simulink model "invPen_PID_LQR"  (R2018b)
settings: Solver=VariableStepAuto  StartTime=0.0  StopTime=20  RelTol=1e-3
libraries: simulink x4
settings Model: Creator=刘越千  LastModifiedBy=刘越千

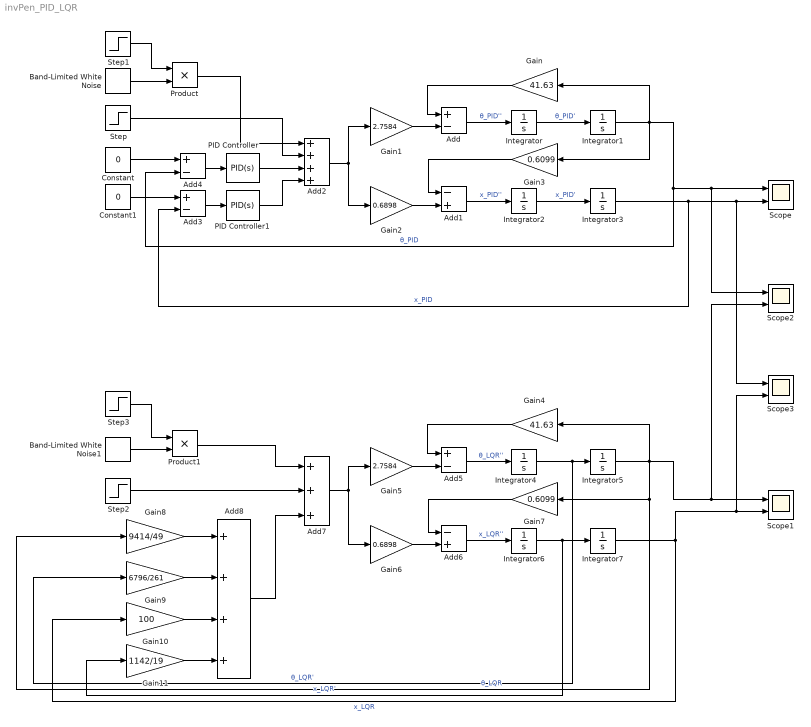
== system invPen_PID_LQR ==
  Add{,3..5} (4 alike) : Sum  Inputs=+-
  Add1 : Sum  Inputs=-+
  Add2 : Sum  Inputs=++++
  Add6 : Sum  Inputs=-+
  Add7 : Sum  Inputs=+++
  Add8 : Sum  Inputs=++++
  Band-Limited White Noise : simulink/Sources/Band-Limited White Noise  Cov=0.1  Ts=0.1  seed=[23341]
  Band-Limited White Noise1 : simulink/Sources/Band-Limited White Noise  Cov=0.1  Ts=0.1  seed=[23341]
  Constant : Constant  Value=0
  Constant1 : Constant  Value=0
  Gain : Gain  Gain=41.63
  Gain1 : Gain  Gain=2.7584
  Gain10 : Gain  Gain=100
  Gain11 : Gain  Gain=1142/19
  Gain2 : Gain  Gain=0.6898
  Gain3 : Gain  Gain=0.6099
  Gain4 : Gain  Gain=41.63
  Gain5 : Gain  Gain=2.7584
  Gain6 : Gain  Gain=0.6898
  Gain7 : Gain  Gain=0.6099
  Gain8 : Gain  Gain=9414/49
  Gain9 : Gain  Gain=6796/261
  Integrator{,2..4,6..7} (6 alike) : Integrator
  Integrator1 : Integrator  InitialCondition=0.1
  Integrator5 : Integrator  InitialCondition=0.1
  PID Controller : simulink/Continuous/PID Controller  Controller=PID  Form=Parallel  TimeDomain=Continuous-time  SampleTime=-1  IntegratorMethod=Forward Euler  FilterMethod=Forward Euler  ControllerParametersSource=internal  P=-321.380817906765  I=-1035.04229145538  D=-24.5033293148827  UseFilter=on  N=375.204412983525  TunerSelectOption=Transfer Function Based (PID Tuner App)  InitialConditionSource=internal  InitialConditionForIntegrator=0  InitialConditionForFilter=0  DifferentiatorICPrevScaledInput=0  ExternalReset=none  TrackingMode=off  Kt=1  LimitOutput=off  UpperSaturationLimit=inf  LowerSaturationLimit=-inf  LinearizeAsGain=on  AntiWindupMode=none  Kb=1  POutMin=[]  POutMax=[]  IOutMin=[]  IOutMax=[]  DOutMin=[]  DOutMax=[]  NOutMin=[]  NOutMax=[]  SumOutMin=[]  SumOutMax=[]  SaturationOutMin=[]  SaturationOutMax=[]  PParamMin=[]  PParamMax=[]  IParamMin=[]  IParamMax=[]  DParamMin=[]  DParamMax=[]  NParamMin=[]  NParamMax=[]  KbParamMin=[]  KbParamMax=[]  KtParamMin=[]  KtParamMax=[]  KbOutMin=[]  KbOutMax=[]  KtOutMin=[]  KtOutMax=[]  IntegratorOutMin=[]  IntegratorOutMax=[]  FilterOutMin=[]  FilterOutMax=[]  SumI1OutMin=[]  SumI1OutMax=[]  SumI2OutMin=[]  SumI2OutMax=[]  SumI3OutMin=[]  SumI3OutMax=[]  SumI4OutMin=[]  SumI4OutMax=[]  SumDOutMin=[]  SumDOutMax=[]  DifferentiatorOutMin=[]  DifferentiatorOutMax=[]  FilterDiffOutCoefMin=[]  FilterDiffOutCoefMax=[]  ReciprocalOutMin=[]  ReciprocalOutMax=[]  SumDenOutMin=[]  SumDenOutMax=[]  SumNumOutMin=[]  SumNumOutMax=[]  DivideOutMin=[]  DivideOutMax=[]  IntegratorContinuousStateAttributes=''  IntegratorStateMustResolveToSignalObject=off  IntegratorRTWStateStorageClass=Auto  FilterContinuousStateAttributes=''  FilterStateMustResolveToSignalObject=off  FilterRTWStateStorageClass=Auto  ParallelPVariant=InternalParameters  IdealPVariant=Disabled  IVariant=InternalParameters  DVariant=InternalParameters  IntegratorVariant=Continuous  SatVariant=Disabled  AWVariant=Passthrough  PCopyVariant=Disabled  TRVariant=Disabled  FdbkBlocksVariant=Forward  IdealPFdbkVariant=Disabled  SatFdbkVariant=Disabled  DerivativeFilterVariant=ContFilter  NVariant=InternalParameters  NCopyVariant=Disabled  FilterICVariant=InternalICsFilter  IntegratorICVariant=InternalICs  ExternalResetVariant=Disabled  TRSumVariant=Passthrough  SumFdbkVariant=Disabled  SumVariant=Sum_PID
  PID Controller1 : simulink/Continuous/PID Controller  Controller=PID  Form=Parallel  TimeDomain=Continuous-time  SampleTime=-1  IntegratorMethod=Forward Euler  FilterMethod=Forward Euler  ControllerParametersSource=internal  P=-241.711059697562  I=-56.8003532909081  D=-30.0841184690224  UseFilter=on  N=13.870046438424  TunerSelectOption=Transfer Function Based (PID Tuner App)  InitialConditionSource=internal  InitialConditionForIntegrator=0  InitialConditionForFilter=0  DifferentiatorICPrevScaledInput=0  ExternalReset=none  TrackingMode=off  Kt=1  LimitOutput=off  UpperSaturationLimit=inf  LowerSaturationLimit=-inf  LinearizeAsGain=on  AntiWindupMode=none  Kb=1  POutMin=[]  POutMax=[]  IOutMin=[]  IOutMax=[]  DOutMin=[]  DOutMax=[]  NOutMin=[]  NOutMax=[]  SumOutMin=[]  SumOutMax=[]  SaturationOutMin=[]  SaturationOutMax=[]  PParamMin=[]  PParamMax=[]  IParamMin=[]  IParamMax=[]  DParamMin=[]  DParamMax=[]  NParamMin=[]  NParamMax=[]  KbParamMin=[]  KbParamMax=[]  KtParamMin=[]  KtParamMax=[]  KbOutMin=[]  KbOutMax=[]  KtOutMin=[]  KtOutMax=[]  IntegratorOutMin=[]  IntegratorOutMax=[]  FilterOutMin=[]  FilterOutMax=[]  SumI1OutMin=[]  SumI1OutMax=[]  SumI2OutMin=[]  SumI2OutMax=[]  SumI3OutMin=[]  SumI3OutMax=[]  SumI4OutMin=[]  SumI4OutMax=[]  SumDOutMin=[]  SumDOutMax=[]  DifferentiatorOutMin=[]  DifferentiatorOutMax=[]  FilterDiffOutCoefMin=[]  FilterDiffOutCoefMax=[]  ReciprocalOutMin=[]  ReciprocalOutMax=[]  SumDenOutMin=[]  SumDenOutMax=[]  SumNumOutMin=[]  SumNumOutMax=[]  DivideOutMin=[]  DivideOutMax=[]  IntegratorContinuousStateAttributes=''  IntegratorStateMustResolveToSignalObject=off  IntegratorRTWStateStorageClass=Auto  FilterContinuousStateAttributes=''  FilterStateMustResolveToSignalObject=off  FilterRTWStateStorageClass=Auto  ParallelPVariant=InternalParameters  IdealPVariant=Disabled  IVariant=InternalParameters  DVariant=InternalParameters  IntegratorVariant=Continuous  SatVariant=Disabled  AWVariant=Passthrough  PCopyVariant=Disabled  TRVariant=Disabled  FdbkBlocksVariant=Forward  IdealPFdbkVariant=Disabled  SatFdbkVariant=Disabled  DerivativeFilterVariant=ContFilter  NVariant=InternalParameters  NCopyVariant=Disabled  FilterICVariant=InternalICsFilter  IntegratorICVariant=InternalICs  ExternalResetVariant=Disabled  TRSumVariant=Passthrough  SumFdbkVariant=Disabled  SumVariant=Sum_PID
  Product : Product
  Product1 : Product
  Scope{,1..3} (4 alike) : Scope  NumInputPorts=2
  Step : Step  Time=2  After=10  SampleTime=0
  Step1 : Step  Time=15  SampleTime=0
  Step2 : Step  Time=2  After=10  SampleTime=0
  Step3 : Step  Time=15  SampleTime=0
  wires:
  Gain11/1 -> Add8/4
  Band-Limited White Noise1/1 -> Product1/2
  Integrator7/1 -> Gain10/1, Scope3/2, Scope1/2  "x_LQR"
  Gain6/1 -> Add6/2
  Step3/1 -> Product1/1
  Add7/1 -> Gain6/1, Gain5/1
  Add8/1 -> Add7/3
  Integrator6/1 -> Gain11/1, Integrator7/1  "x_LQR'"
  Integrator5/1 -> Gain8/1, Gain7/1, Scope2/2, Scope1/1, Gain4/1  "θ_LQR"
  Gain10/1 -> Add8/3
  Gain4/1 -> Add5/1
  Step2/1 -> Add7/2
  Gain8/1 -> Add8/1
  Add6/1 -> Integrator6/1  "x_LQR''"
  Add5/1 -> Integrator4/1  "θ_LQR''"
  Integrator4/1 -> Gain9/1, Integrator5/1  "θ_LQR'"
  Gain9/1 -> Add8/2
  Product1/1 -> Add7/1
  Gain7/1 -> Add6/1
  Gain5/1 -> Add5/2
  Step1/1 -> Product/1
  Band-Limited White Noise/1 -> Product/2
  Product/1 -> Add2/1
  Constant1/1 -> Add3/1
  PID Controller/1 -> Add2/3
  Add3/1 -> PID Controller1/1
  Gain/1 -> Add/1
  PID Controller1/1 -> Add2/4
  Add/1 -> Integrator/1  "θ_PID''"
  Integrator3/1 -> Add3/2, Scope3/1, Scope/2  "x_PID"
  Integrator2/1 -> Integrator3/1  "x_PID'"
  Add4/1 -> PID Controller/1
  Add1/1 -> Integrator2/1  "x_PID''"
  Gain2/1 -> Add1/2
  Step/1 -> Add2/2
  Gain3/1 -> Add1/1
  Constant/1 -> Add4/1
  Integrator1/1 -> Gain3/1, Scope2/1, Scope/1, Add4/2, Gain/1  "θ_PID"
  Gain1/1 -> Add/2
  Add2/1 -> Gain2/1, Gain1/1
  Integrator/1 -> Integrator1/1  "θ_PID'"
